simulink model "line_following_algorithm_autosave"  (R2019b)
settings: Solver=FixedStepDiscrete  StartTime=0.0  StopTime=1600  FixedStep=0.01  RelTol=1e-3
values from neighbouring files (symbols this model uses):
  initial_theta = 0    [main_script.m]    (also in variables.mat)
  initial_x = 0.5801    [main_script.m]    (also in variables.mat)
  initial_y = 0.4825    [main_script.m]    (also in variables.mat)
  lineLength = 0.666666666667    [variables.mat]
  mapForSim =     [Line_Following_Map.mat]    (also in variables.mat)
  xcor_max = xcor_max_list(aisle_num)    [aisle_branch.m]    (also in variables.mat = 5.65)
  xcor_min = xcor_min_list(aisle_num)    [aisle_branch.m]    (also in variables.mat = 5.6)
  ycor_max = ycor_max_list(aisle_num)    [aisle_branch.m]    (also in variables.mat = 3.5)
  ycor_min = ycor_min_list(aisle_num)    [aisle_branch.m]    (also in variables.mat = 3.45)
undefined symbols (not defined in the file or in its folder): DiscIntNeverNeededParam
libraries: mobileRoboticsTrainingLib x3
settings Model: Creator=Owner  LastModifiedBy=Owner

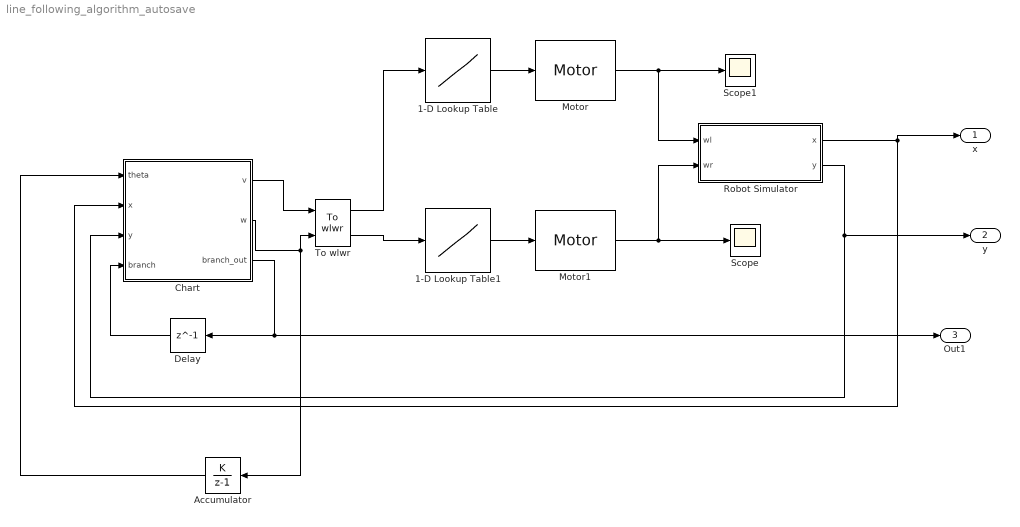
== system line_following_algorithm_autosave ==
  1-D Lookup Table : Lookup_n-D  NumberOfTableDimensions=1  BreakpointsForDimension1=[-5:5]  Table=tanh([-5:5])  InternalRulePriority=Speed  RndMeth=Simplest  InputSameDT=on
  1-D Lookup Table1 : Lookup_n-D  NumberOfTableDimensions=1  BreakpointsForDimension1=[-5:5]  Table=tanh([-5:5])  InternalRulePriority=Speed  RndMeth=Simplest  InputSameDT=on
  Accumulator : DiscreteIntegrator  IntegratorMethod=Accumulation: Forward Euler  SampleTime=-1  ICPrevOutput=DiscIntNeverNeededParam  ICPrevScaledInput=DiscIntNeverNeededParam
  Chart : Stateflow chart  BlockKeywords=__PRM__SERIALIZED__DATA__:Stateflow Chart,Stateflow Diagram  TreatAsAtomicUnit=on
  Delay : Delay  DelayLength=1  InitialCondition=0
  Motor : mobileRoboticsTrainingLib/Motor  motorPlant=1  sensorType=Speed
      settings: SourceProductName=Mobile Robotics Training Library
  Motor1 : mobileRoboticsTrainingLib/Motor  motorPlant=1  sensorType=Speed
      settings: SourceProductName=Mobile Robotics Training Library
  Robot Simulator : Subsystem  Priority=99  AncestorBlock=mobileRoboticsTrainingLib/Robot Simulator  mask(Robot Simulator){mapVar=mapForSim, startX=initial_x, startY=initial_y, startTheta=initial_theta, axleLength=0.1, wheelR=0.05}
      mask prompts: mapVar "Map Variable"; startX "Start X (m)"; startY "Start Y (m)"; startTheta "Theta (deg)"; axleLength "Axle Length (m)"; wheelR "Wheel Radius (m)"
      mask help: Configure robot simulator to use custom simulation maps and simulate closed-loop mobile robotics systems along with appropriate sensor simulation blocks.
      mask init:
      | set_param(bdroot,'SolverType','Fixed-Step');
      | set_param(bdroot,'Solver','FixedStepDiscrete');
      | 
      | if (exist('Ts'))
      |     set_param(bdroot,'FixedStep','Ts');
      | else
      |     set_param(bdroot,'FixedStep','0.01');
      | end
      | 
      | h = findobj('Name','Robot Simulator');
      | if ~isempty(h)
      |     close (h);
      | end
      | setupRobotSim();
      mask Help: web('Robot Simulator.htm')
      mask DialogControl mapCont Prompt: Map Setup
      mask DialogControl initPosCont Prompt: Initial Position
      mask DialogControl setPos Prompt: Set position interactively
      mask DialogControl setPos Callback:
      | %% Set starting point
      | setStartingPoint();
      mask DialogControl initOrientation Prompt: Initial Orientation
      mask DialogControl robotCharCont Prompt: Robot Characteristics
      mask Display: disp('Robot Simulator')
  Scope : Scope
  Scope1 : Scope
  To wlwr : mobileRoboticsTrainingLib/To wlwr  axleLength=0.1  wheelR=0.05
  x : Outport
  y : Outport  Port=2
  Out1 : Outport  Port=3
  wires:
  To wlwr/2 -> 1-D Lookup Table1/1
  To wlwr/1 -> 1-D Lookup Table/1
  1-D Lookup Table/1 -> Motor/1
  1-D Lookup Table1/1 -> Motor1/1
  Motor/1 -> Scope1/1, Robot Simulator/1(wl)
  Motor1/1 -> Scope/1, Robot Simulator/2(wr)
  Chart/1(v) -> To wlwr/1
  Chart/2(w) -> To wlwr/2, Accumulator/1
  Accumulator/1 -> Chart/1(theta)
  Robot Simulator/2("y ") -> y/1, Chart/3(y)
  Robot Simulator/1("x ") -> x/1, Chart/2(x)
  Chart/3(branch_out) -> Delay/1, Out1/1
  Delay/1 -> Chart/4(branch)

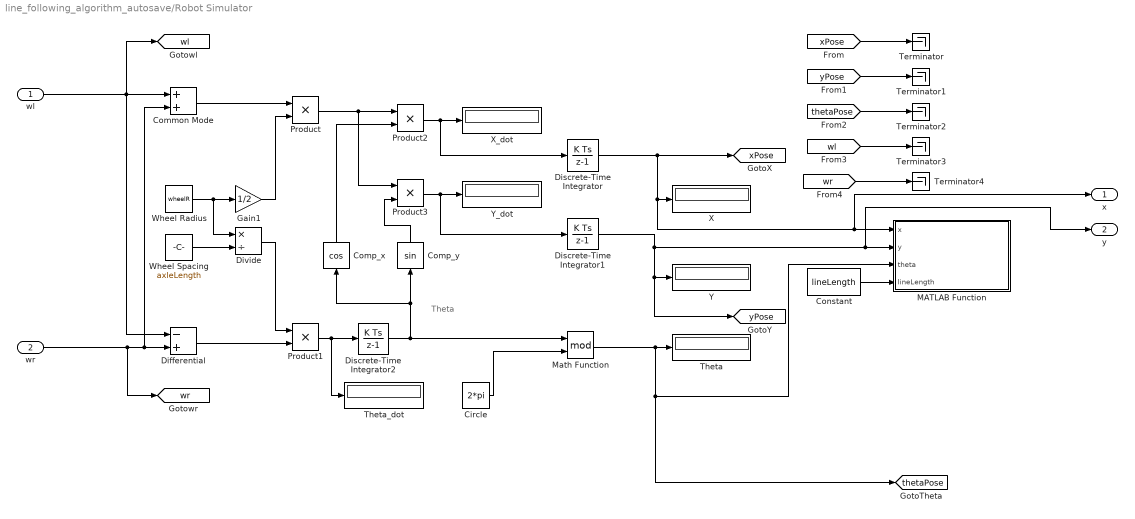
== system line_following_algorithm_autosave/Robot Simulator ==
  note: Theta
  wl : Inport
  wr : Inport  Port=2
  Circle : Constant  Value=2*pi
  Common Mode : Sum
  Comp_x : Trigonometry  Operator=cos
  Comp_y : Trigonometry
  Constant : Constant  Value=lineLength
  Differential : Sum  Inputs=-+
  Discrete-Time Integrator : DiscreteIntegrator  InitialCondition=startX  SampleTime=-1  ICPrevOutput=DiscIntNeverNeededParam  ICPrevScaledInput=DiscIntNeverNeededParam
  Discrete-Time Integrator1 : DiscreteIntegrator  InitialCondition=startY  SampleTime=-1  ICPrevOutput=DiscIntNeverNeededParam  ICPrevScaledInput=DiscIntNeverNeededParam
  Discrete-Time Integrator2 : DiscreteIntegrator  InitialCondition=startTheta*(pi/180)  SampleTime=-1  ICPrevOutput=DiscIntNeverNeededParam  ICPrevScaledInput=DiscIntNeverNeededParam
  Divide : Product  Inputs=*/
  Gain1 : Gain  Gain=1/2
  MATLAB Function : MATLAB Function  TreatAsAtomicUnit=on
  Math Function : Math  Operator=mod  SaturateOnIntegerOverflow=on
  Product{,1..3} (4 alike) : Product  RndMeth=Zero
  Terminator{,1..4} (5 alike) : Terminator
  Theta : Display
  Theta_dot : Display
  Wheel Radius : Constant  Value=wheelR
  Wheel Spacing : Constant  Value=axleLength
  X : Display
  X_dot : Display
  Y : Display
  Y_dot : Display
  "x " : Outport
  "y " : Outport  Port=2
  tag scope: thetaPose=global, wl=global, wr=global, xPose=global, yPose=global
  wires:
  [wr] -> Terminator4/1
  [wl] -> Terminator3/1
  Math Function/1 -> [thetaPose], MATLAB Function/3(theta), Theta/1
  Differential/1 -> Product1/2
  Comp_y/1 -> Product3/2
  Discrete-Time Integrator/1 -> [xPose], "x "/1, MATLAB Function/1(x), X/1
  Product3/1 -> Discrete-Time Integrator1/1, Y_dot/1
  Discrete-Time Integrator1/1 -> Y/1, [yPose], "y "/1, MATLAB Function/2(y)
  Divide/1 -> Product1/1
  wr/1 -> [wr], Common Mode/2, Differential/2
  Discrete-Time Integrator2/1 -> Math Function/1, Comp_x/1, Comp_y/1
  wl/1 -> [wl], Common Mode/1, Differential/1
  Comp_x/1 -> Product2/2
  Product1/1 -> Discrete-Time Integrator2/1, Theta_dot/1
  Wheel Radius/1 -> Divide/1, Gain1/1
  Wheel Spacing/1 -> Divide/2
  Product2/1 -> Discrete-Time Integrator/1, X_dot/1
  Gain1/1 -> Product/2
  Common Mode/1 -> Product/1
  Product/1 -> Product3/1, Product2/1
  Circle/1 -> Math Function/2
  Constant/1 -> MATLAB Function/4(lineLength)
  [xPose] -> Terminator/1
  [yPose] -> Terminator1/1
  [thetaPose] -> Terminator2/1

== matlab function line_following_algorithm_autosave/Robot Simulator/MATLAB Function ==
  data: x input; y input; theta input; lineLength input
function plotRobot(x,y,theta,lineLength)
% Get plot details
coder.extrinsic('evalin','plot')
ph1 = evalin('base','PlotHandle1');
ph2 = evalin('base','PlotHandle2');

% Find length orientation line
xp = [x x+lineLength*cos(theta)];
yp = [y y+lineLength*sin(theta)];

% Plot robot
set(ph1,'xdata',xp,'ydata',yp);
set(ph2,'xdata',x,'ydata',y);
drawnow('limitrate')

== stateflow chart line_following_algorithm_autosave/Chart ==
  state Move_to_top_aisle
    entry: v = 0.01
    w = 0;
    top = 1;
    bottom = 0;
  state Obstacle_detection_stop
    entry: v = 0;
    w = 0;
  state Forward
    entry: v = 0.01;
    w = 0;
    branch_out = 1
  state Reverse_to_bottom_aisle
    entry: v = -0.01;
    w = 0;
    bottom = 1;
    top = 0;
  state Reverse
    entry: v = -0.01;
    w = 0;
    branch_out = 1;
  state Initial
    entry: v = 0;
    w = 0;
    right = 0;
    left = 0;
    arrived = 0;
  state RightLeft
    entry: right = 1;
    left = 0;
    bottom = 1;
    top = 0;
  state Stop_at_aisle
    entry: v = 0;
    w = 0;
    branch_out = 0;
    current_theta = theta;
  state GoStraightAisle
    entry: v = 0.01;
    w = 0;
    current_theta = theta
  state Stop_at_station
    entry: v =0;
    w = 0;
    arrived = 1
  state Turn90CCtoAisle
    entry: v = 0;
    w = 0.2;
    branch_out = 0
    right = 0;
    left = 1;
  state Turn90CtoAisle
    entry: v = 0;
    w = -0.2;
    left = 0;
    right = 1;
    branch_out = 0;
  state Turn90CCtoBranch
    entry: v = 0;
    w = 0.2;
    branch_out = 1;
  state Turn90CBranch
    entry: v = 0;
    w = -0.2;
    branch_out = 1;
  state Stop_oriented
    entry: v = 0;
    w = 0;
  (default) -> Initial
  Initial -> Move_to_top_aisle [order 5] : [x>xcor_max & y > 3 | x<xcor_min & y > 3]
  GoStraightAisle -> Obstacle_detection_stop [order 4] : [x>xcor_min & x < xcor_max & y> ycor_min_o-0.3]
  Initial -> Forward [order 3] : [y< ycor_min & x < xcor_max & x>=xcor_min]
  Forward -> Stop_at_station : [y>=ycor_min & y < ycor_max]
  Initial -> Reverse_to_bottom_aisle [order 4] : [x>xcor_max & y < 3 | x<xcor_min & y < 3]
  Initial -> Reverse [order 2] : [ y>ycor_max & x<xcor_max & x>=xcor_min]
  Reverse_to_bottom_aisle -> Stop_at_aisle : [y<0.5 & y >=0.47]
  Turn90CCtoBranch -> Reverse [order 2] : [theta >= current_theta+205 & theta <current_theta+207 & top]
  Turn90CBranch -> Reverse [order 2] : [theta <= current_theta-205 & top ]
  Reverse -> Stop_at_station : [y >ycor_min & y <= ycor_max]
  Initial -> RightLeft [order 1] : [x == 0.5801 & y == 0.4825]
  RightLeft -> GoStraightAisle
  GoStraightAisle -> Stop_at_station [order 2] : [y >= ycor_min & y < ycor_max & branch]
  Stop_at_aisle -> GoStraightAisle [order 3] : [theta <= current_theta+ 205 & x < xcor_min]
  Stop_at_aisle -> Turn90CCtoAisle [order 1] : [x > xcor_max]
  Turn90CCtoAisle -> GoStraightAisle : [theta >= current_theta+205 & theta <current_theta+207]
  Stop_at_aisle -> Turn90CtoAisle [order 2] : [x < xcor_min]
  Stop_oriented -> GoStraightAisle
  GoStraightAisle -> Turn90CCtoBranch [order 1] : [x >= xcor_min & x < xcor_max & ~branch & right]
  Turn90CCtoBranch -> GoStraightAisle [order 1] : [theta >= current_theta+205 & theta <current_theta+207 & bottom]
  GoStraightAisle -> Turn90CBranch [order 3] : [(x >= xcor_min & x < xcor_max & ~branch & left)]
  Turn90CBranch -> GoStraightAisle [order 1] : [theta <= current_theta-205 & bottom]
  Turn90CtoAisle -> Stop_oriented : [theta<=current_theta-205]
  data: theta input; x input; y input; v output; w output; xcor_max parameter; xcor_min parameter; ycor_max parameter; ycor_min parameter; branch_out output; current_theta local; right local; left local; bottom local; top local; arrived local; branch input; ycor_min_o local
